simulink model "nonlinsim"  (R2024b)
settings: Solver=ode45  StartTime=tspan(1)  StopTime=tspan(2)  RelTol=1e-3
values from neighbouring files (symbols this model uses):
  b = dtf.num    [DBReg.m]    (also in disc.m = 2; main.m = 2)
  J = 0.5    [disc.m]    (also in main.m)
  k = 1    [disc.m]    (also in main.m)
  PSDNaslinReg = PSD(NaslinReg, Ts_reg)    [main.m]
  Ts = 0.5    [disc.m]    (also in main.m = 0.475)
settings Model: Creator=markminerov  LastModifiedBy=markminerov

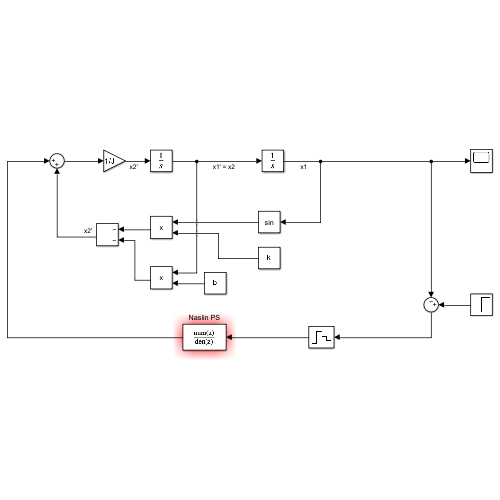
[thumbnail: Simulink's stored preview of the top-level diagram]
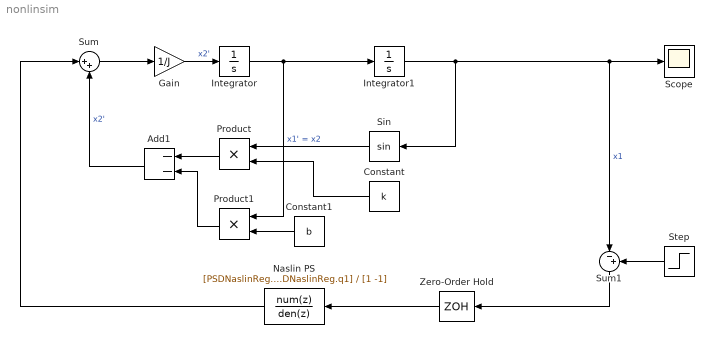
== system nonlinsim ==
  Add1 : Sum  Inputs=--
  Constant : Constant  Value=k
  Constant1 : Constant  Value=b
  Gain : Gain  Gain=1/J
  Integrator : Integrator
  Integrator1 : Integrator
  Naslin PS : DiscreteTransferFcn  Numerator=[PSDNaslinReg.q0 PSDNaslinReg.q1]  Denominator=[1 -1]
  Product : Product
  Product1 : Product
  Scope : Scope
  Sin : Trigonometry
  Step : Step  After=u  SampleTime=0
  Sum : Sum  Inputs=|++
  Sum1 : Sum  Inputs=|-+
  Zero-Order Hold : ZeroOrderHold  SampleTime=Ts
  wires:
  Integrator/1 -> Integrator1/1, Product1/1  "x1' = x2"
  Integrator1/1 -> Sin/1, Sum1/1, Scope/1  "x1"
  Sin/1 -> Product/1
  Constant/1 -> Product/2
  Product/1 -> Add1/1
  Constant1/1 -> Product1/2
  Product1/1 -> Add1/2
  Gain/1 -> Integrator/1  "x2'"
  Add1/1 -> Sum/2  "x2'"
  Sum/1 -> Gain/1
  Step/1 -> Sum1/2
  Zero-Order Hold/1 -> Naslin PS/1
  Sum1/1 -> Zero-Order Hold/1
  Naslin PS/1 -> Sum/1
